simulink model "Bicycle_model_Steady_State"  (R2022b)
settings: Solver=FixedStepAuto  StartTime=0.0  StopTime=40  FixedStep=0.01  RelTol=1e-3
values from neighbouring files (symbols this model uses):
  a = 1.8    [Bicycle_model_parameters_formula.m]    (also in Bicycle_model_parameters_road_vehicle.m = 1.1)
  A = 1.25    [Bicycle_model_parameters_formula.m]    (also in Bicycle_model_parameters_road_vehicle.m = 1.8)
  a1f = -1e-5    (= -1e-05)    [Bicycle_model_parameters_formula.m]    (also in Bicycle_model_parameters_road_vehicle.m)
  a1r = -1e-5    (= -1e-05)    [Bicycle_model_parameters_formula.m]    (also in Bicycle_model_parameters_road_vehicle.m)
  a2f = 1.25    [Bicycle_model_parameters_formula.m]    (also in Bicycle_model_parameters_road_vehicle.m = 0.95)
  a2r = 1.25    [Bicycle_model_parameters_formula.m]    (also in Bicycle_model_parameters_road_vehicle.m = 0.95)
  b = L-a    (= 1.7)    [Bicycle_model_parameters_formula.m]    (also in Bicycle_model_parameters_road_vehicle.m)
  Bf = 0.2719    [Bicycle_model_parameters_formula.m]    (also in Bicycle_model_parameters_road_vehicle.m = 0.0813)
  Br = 0.3609    [Bicycle_model_parameters_formula.m]    (also in Bicycle_model_parameters_road_vehicle.m = 0.0925)
  Cf = 1.8391    [Bicycle_model_parameters_formula.m]    (also in Bicycle_model_parameters_road_vehicle.m = 1.2947)
  Cr = 1.7631    [Bicycle_model_parameters_formula.m]    (also in Bicycle_model_parameters_road_vehicle.m = 1.2617)
  cz = 1    [Bicycle_model_parameters_formula.m]    (also in Bicycle_model_parameters_road_vehicle.m = 0)
  Ef = -2.5276    [Bicycle_model_parameters_formula.m]    (also in Bicycle_model_parameters_road_vehicle.m = -8.3966)
  Er = -1.989    [Bicycle_model_parameters_formula.m]    (also in Bicycle_model_parameters_road_vehicle.m = -8.7012)
  g = 9.81    [Bicycle_model_parameters_formula.m]    (also in Bicycle_model_parameters_road_vehicle.m)
  I = 1500    [Bicycle_model_parameters_formula.m]    (also in Bicycle_model_parameters_road_vehicle.m = 3500)
  L = 3.5    [Bicycle_model_parameters_formula.m]    (also in Bicycle_model_parameters_road_vehicle.m = 2.8)
  m = 850    [Bicycle_model_parameters_formula.m]    (also in Bicycle_model_parameters_road_vehicle.m = 1650)
  rho = 1.225    [Bicycle_model_parameters_formula.m]    (also in Bicycle_model_parameters_road_vehicle.m)
  SR = 10    [Bicycle_model_parameters_formula.m]    (also in Bicycle_model_parameters_road_vehicle.m = 20)
libraries: simulink_extras x5, simulink x1
settings Model: Creator=webstert  LastModifiedBy=webstert

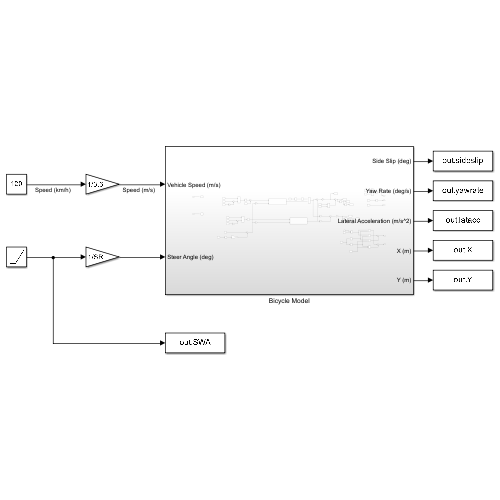
[thumbnail: Simulink's stored preview of the top-level diagram]
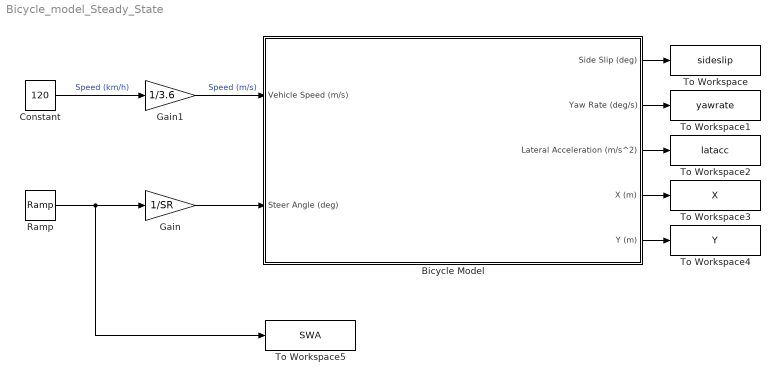
== system Bicycle_model_Steady_State ==
  Bicycle Model : Subsystem
  Constant : Constant  Value=120
  Gain : Gain  Gain=1/SR
  Gain1 : Gain  Gain=1/3.6
  Ramp : simulink/Sources/Ramp  slope=2  start=0  InitialOutput=0
  To Workspace : ToWorkspace  VariableName=sideslip  SaveFormat=Timeseries  SampleTime=-1
  To Workspace1 : ToWorkspace  VariableName=yawrate  SaveFormat=Timeseries  SampleTime=-1
  To Workspace2 : ToWorkspace  VariableName=latacc  SaveFormat=Timeseries  SampleTime=-1
  To Workspace3 : ToWorkspace  VariableName=X  SaveFormat=Timeseries  SampleTime=-1
  To Workspace4 : ToWorkspace  VariableName=Y  SaveFormat=Timeseries  SampleTime=-1
  To Workspace5 : ToWorkspace  VariableName=SWA  SaveFormat=Timeseries  SampleTime=-1
  wires:
  Bicycle Model/1(Side Slip (deg)) -> To Workspace/1
  Bicycle Model/2(Yaw Rate (deg/s)) -> To Workspace1/1
  Bicycle Model/3(Lateral Acceleration (m/s^2)) -> To Workspace2/1
  Bicycle Model/4(X (m)) -> To Workspace3/1
  Bicycle Model/5(Y (m)) -> To Workspace4/1
  Gain/1 -> Bicycle Model/2(Steer Angle (deg))
  Constant/1 -> Gain1/1  "Speed (km/h)"
  Gain1/1 -> Bicycle Model/1(Vehicle Speed (m/s))  "Speed (m/s)"
  Ramp/1 -> To Workspace5/1, Gain/1

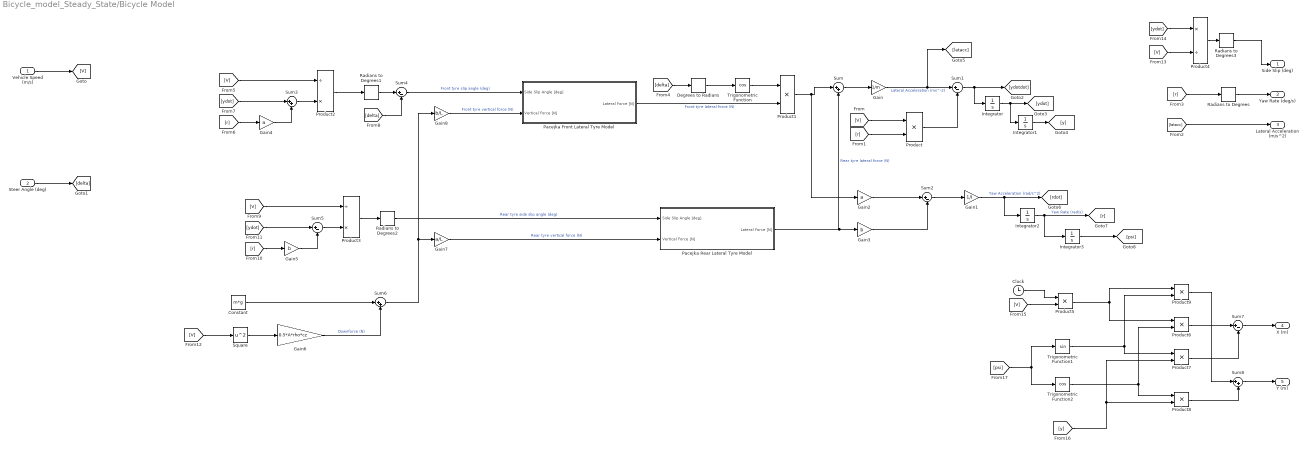
== system Bicycle_model_Steady_State/Bicycle Model ==
  Vehicle Speed (m/s) : Inport
  Steer Angle (deg) : Inport  Port=2
  Clock : Clock
  Constant : Constant  Value=m*g
  Degrees to Radians : simulink_extras/Transformations/Degrees to Radians
  Gain : Gain  Gain=1/m
  Gain1 : Gain  Gain=1/I
  Gain2 : Gain  Gain=a
  Gain3 : Gain  Gain=b
  Gain4 : Gain  Gain=a
  Gain5 : Gain  Gain=b
  Gain6 : Gain  Gain=0.5*A*rho*cz
  Gain7 : Gain  Gain=a/L
  Gain8 : Gain  Gain=b/L
  Integrator{,1..3} (4 alike) : Integrator
  Pacejka Front Lateral Tyre Model : Subsystem
  Pacejka Rear Lateral Tyre Model : Subsystem
  Product{,1,5..9} (7 alike) : Product
  Product2 : Product  Inputs=/*
  Product3 : Product  Inputs=/*
  Product4 : Product  Inputs=*/
  Radians to Degrees{,1..3} (4 alike) : simulink_extras/Transformations/Radians to Degrees
  Square : Math  Operator=square
  Sum{,3,6,8} (4 alike) : Sum  Inputs=|++
  Sum{1..2,4..5,7} (5 alike) : Sum  Inputs=|+-
  Trigonometric Function : Trigonometry  Operator=cos
  Trigonometric Function1 : Trigonometry
  Trigonometric Function2 : Trigonometry  Operator=cos
  Side Slip (deg) : Outport
  Yaw Rate (deg/s) : Outport  Port=2
  Lateral Acceleration (m/s^2) : Outport  Port=3
  X (m) : Outport  Port=4
  Y (m) : Outport  Port=5
  wires:
  Vehicle Speed (m/s)/1 -> [V]
  Steer Angle (deg)/1 -> [delta]
  Sum/1 -> Gain/1
  Gain/1 -> [latacc], Sum1/1  "Lateral Acceleration (ms^-2)"
  Product/1 -> Sum1/2
  [V] -> Product/1
  [r] -> Product/2
  Sum1/1 -> Integrator/1, [ydotdot]
  Integrator/1 -> Integrator1/1, [ydot]
  Integrator1/1 -> [y]
  [latacc] -> Lateral Acceleration (m/s^2)/1
  Sum2/1 -> Gain1/1
  Gain1/1 -> Integrator2/1, [rdot]  "Yaw Acceleration (rad/s^2)"
  Integrator2/1 -> Integrator3/1, [r]  "Yaw Rate (rad/s)"
  Integrator3/1 -> [psi]
  [r] -> Radians to Degrees/1
  Radians to Degrees/1 -> Yaw Rate (deg/s)/1
  Gain2/1 -> Sum2/1
  Gain3/1 -> Sum2/2
  Pacejka Rear Lateral Tyre Model/1(Lateral Force [N]) -> Sum/2, Gain3/1  "Rear tyre lateral force (N)"
  Pacejka Front Lateral Tyre Model/1(Lateral Force [N]) -> Product1/2  "Front tyre lateral force (N)"
  [delta] -> Degrees to Radians/1
  Product1/1 -> Gain2/1, Sum/1
  Degrees to Radians/1 -> Trigonometric Function/1
  Trigonometric Function/1 -> Product1/1
  [r] -> Gain4/1
  [ydot] -> Sum3/1
  Gain4/1 -> Sum3/2
  [V] -> Product2/1
  Sum3/1 -> Product2/2
  Product2/1 -> Radians to Degrees1/1
  Radians to Degrees1/1 -> Sum4/1
  [delta] -> Sum4/2
  Sum4/1 -> Pacejka Front Lateral Tyre Model/1(Side Slip Angle [deg])  "Front tyre slip angle (deg)"
  Product3/1 -> Radians to Degrees2/1
  Sum5/1 -> Product3/2
  [V] -> Product3/1
  Gain5/1 -> Sum5/2
  [ydot] -> Sum5/1
  [r] -> Gain5/1
  Radians to Degrees2/1 -> Pacejka Rear Lateral Tyre Model/1(Side Slip Angle [deg])  "Rear tyre side slip angle (deg)"
  Constant/1 -> Sum6/1
  [V] -> Square/1
  Gain6/1 -> Sum6/2  "Downforce (N)"
  Square/1 -> Gain6/1
  Sum6/1 -> Gain7/1, Gain8/1
  Gain7/1 -> Pacejka Rear Lateral Tyre Model/2(Vertical Force [N])  "Rear tyre vertical force (N)"
  Gain8/1 -> Pacejka Front Lateral Tyre Model/2(Vertical Force [N])  "Front tyre vertical force (N)"
  [ydot] -> Product4/1
  [V] -> Product4/2
  Product4/1 -> Radians to Degrees3/1
  Radians to Degrees3/1 -> Side Slip (deg)/1
  Clock/1 -> Product5/1
  [V] -> Product5/2
  [psi] -> Trigonometric Function2/1, Trigonometric Function1/1
  Product5/1 -> Product6/1, Product9/1
  Trigonometric Function1/1 -> Product7/1, Product9/2
  Trigonometric Function2/1 -> Product6/2, Product8/1
  [y] -> Product7/2, Product8/2
  Product7/1 -> Sum7/2
  Product6/1 -> Sum7/1
  Sum7/1 -> X (m)/1
  Sum8/1 -> Y (m)/1
  Product9/1 -> Sum8/1
  Product8/1 -> Sum8/2

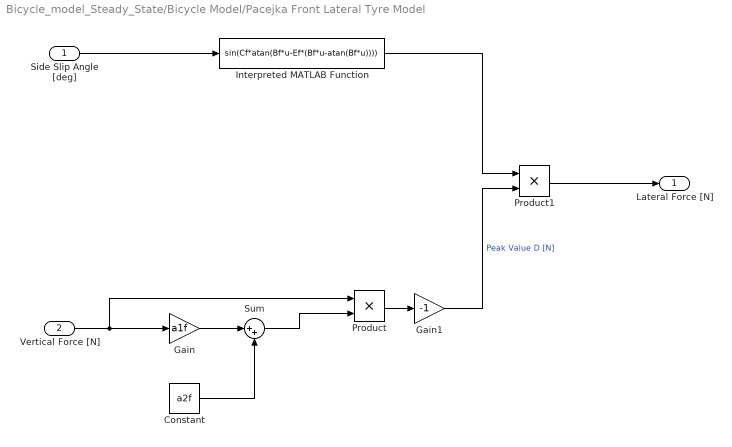
== system Bicycle_model_Steady_State/Bicycle Model/Pacejka Front Lateral Tyre Model ==
  Side Slip Angle [deg] : Inport
  Vertical Force [N] : Inport  Port=2
  Constant : Constant  Value=a2f
  Gain : Gain  Gain=a1f
  Gain1 : Gain  Gain=-1
  Interpreted MATLAB Function : MATLABFcn  MATLABFcn=sin(Cf*atan(Bf*u-Ef*(Bf*u-atan(Bf*u))))
  Product : Product
  Product1 : Product
  Sum : Sum  Inputs=|++
  Lateral Force [N] : Outport
  wires:
  Product1/1 -> Lateral Force [N]/1
  Interpreted MATLAB Function/1 -> Product1/1
  Side Slip Angle [deg]/1 -> Interpreted MATLAB Function/1
  Gain1/1 -> Product1/2  "Peak Value D [N]"
  Product/1 -> Gain1/1
  Sum/1 -> Product/2
  Gain/1 -> Sum/1
  Constant/1 -> Sum/2
  Vertical Force [N]/1 -> Gain/1, Product/1

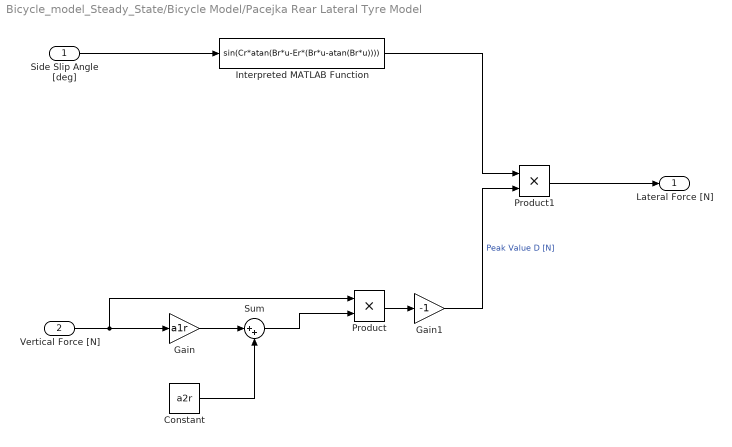
== system Bicycle_model_Steady_State/Bicycle Model/Pacejka Rear Lateral Tyre Model ==
  Side Slip Angle [deg] : Inport
  Vertical Force [N] : Inport  Port=2
  Constant : Constant  Value=a2r
  Gain : Gain  Gain=a1r
  Gain1 : Gain  Gain=-1
  Interpreted MATLAB Function : MATLABFcn  MATLABFcn=sin(Cr*atan(Br*u-Er*(Br*u-atan(Br*u))))
  Product : Product
  Product1 : Product
  Sum : Sum  Inputs=|++
  Lateral Force [N] : Outport
  wires:
  Vertical Force [N]/1 -> Product/1, Gain/1
  Constant/1 -> Sum/2
  Gain/1 -> Sum/1
  Sum/1 -> Product/2
  Product/1 -> Gain1/1
  Gain1/1 -> Product1/2  "Peak Value D [N]"
  Side Slip Angle [deg]/1 -> Interpreted MATLAB Function/1
  Interpreted MATLAB Function/1 -> Product1/1
  Product1/1 -> Lateral Force [N]/1
